simulink model "sm_boom_lift_crawler"  (R2026a)
settings: Solver=ode23t  StopTime=tVec.StopTime  FixedStep=2e-3  MaxStep=2  AbsTol=1e-3
StartFcn:
  | tic;
StopFcn:
  | Elapsed_Sim_Time = toc;
  | %disp(['Elapsed Sim Time = ' num2str(Elapsed_Sim_Time)]);
undefined symbols (not defined in the file): BasketR, Boom, Chassis, Extend, Jib, LevelM, LevelS, Lift, operator_seq, OutFL, OutFR, OutRL, OutRR, oVec, Tilt, TrackL, TrackR, Turret, tVec
libraries: sm_boom_lift_crawler_lib x14, nesl_utility x2, sm_lib x2, sm_boom_lift_crawler_lib_actuators x1, sm_boom_lift_crawler_lib_control x1, sm_boom_lift_crawler_lib_lift x1
(part 2 of 2)

== system sm_boom_lift_crawler/Control/Valve Sequence/Sky Valve Commands/Basket LevelS Selector Valve ==
  t : Inport
  Selector Valve Input : Lookup_n-D  NumberOfTableDimensions=1  BreakpointsForDimension1=[0 1]  Table=[0 0]  InterpMethod=Flat  ExtrapMethod=Clip  UseLastTableValue=on  InternalRulePriority=Speed  RndMeth=Simplest
  C : Outport
  wires:
  t/1 -> Selector Valve Input/1
  Selector Valve Input/1 -> C/1

== system sm_boom_lift_crawler/Control/Valve Sequence/Sky Valve Commands/BasketR Selector Valve (r2) ==
  t : Inport
  Selector Valve Input : Lookup_n-D  NumberOfTableDimensions=1  BreakpointsForDimension1=tVec.sky.r2.all  Table=oVec.sky.r2.all  InterpMethod=Flat  ExtrapMethod=Clip  UseLastTableValue=on  InternalRulePriority=Speed  RndMeth=Simplest
  C : Outport
  wires:
  Selector Valve Input/1 -> C/1
  t/1 -> Selector Valve Input/1

== system sm_boom_lift_crawler/Control/Valve Sequence/Sky Valve Commands/Extend Selector Valve (c3) ==
  t : Inport
  Selector Valve Input : Lookup_n-D  NumberOfTableDimensions=1  BreakpointsForDimension1=tVec.sky.c3.all  Table=oVec.sky.c3.all  InterpMethod=Flat  ExtrapMethod=Clip  UseLastTableValue=on  InternalRulePriority=Speed  RndMeth=Simplest
  C : Outport
  wires:
  t/1 -> Selector Valve Input/1
  Selector Valve Input/1 -> C/1

== system sm_boom_lift_crawler/Control/Valve Sequence/Sky Valve Commands/Jib Selector Valve (c4) ==
  t : Inport
  Selector Valve Input : Lookup_n-D  NumberOfTableDimensions=1  BreakpointsForDimension1=tVec.sky.c4.all  Table=oVec.sky.c4.all  InterpMethod=Flat  ExtrapMethod=Clip  UseLastTableValue=on  InternalRulePriority=Speed  RndMeth=Simplest
  C : Outport
  wires:
  Selector Valve Input/1 -> C/1
  t/1 -> Selector Valve Input/1

== system sm_boom_lift_crawler/Control/Valve Sequence/Sky Valve Commands/Lift Selector Valve (c1) ==
  t : Inport
  Selector Valve Input : Lookup_n-D  NumberOfTableDimensions=1  BreakpointsForDimension1=tVec.sky.c1.all  Table=oVec.sky.c1.all  InterpMethod=Flat  ExtrapMethod=Clip  UseLastTableValue=on  InternalRulePriority=Speed  RndMeth=Simplest
  C : Outport
  wires:
  t/1 -> Selector Valve Input/1
  Selector Valve Input/1 -> C/1

== system sm_boom_lift_crawler/Control/Valve Sequence/Sky Valve Commands/Sky Manifold Proportional Valve ==
  t : Inport
  Selector Valve Input : Lookup_n-D  NumberOfTableDimensions=1  BreakpointsForDimension1=tVec.sky.proportional  Table=oVec.sky.proportional  InterpMethod=Flat  ExtrapMethod=Clip  UseLastTableValue=on  InternalRulePriority=Speed  RndMeth=Simplest
  C : Outport
  wires:
  t/1 -> Selector Valve Input/1
  Selector Valve Input/1 -> C/1

== system sm_boom_lift_crawler/Control/Valve Sequence/Sky Valve Commands/Tilt Selector Valve (c2) ==
  t : Inport
  Selector Valve Input : Lookup_n-D  NumberOfTableDimensions=1  BreakpointsForDimension1=tVec.sky.c2.all  Table=oVec.sky.c2.all  InterpMethod=Flat  ExtrapMethod=Clip  UseLastTableValue=on  InternalRulePriority=Speed  RndMeth=Simplest
  C : Outport
  wires:
  Selector Valve Input/1 -> C/1
  t/1 -> Selector Valve Input/1

== system sm_boom_lift_crawler/Control/Valve Sequence/Sky Valve Commands/Turret Selector Valve (r1) ==
  t : Inport
  Selector Valve Input : Lookup_n-D  NumberOfTableDimensions=1  BreakpointsForDimension1=tVec.sky.r1.all  Table=oVec.sky.r1.all  InterpMethod=Flat  ExtrapMethod=Clip  UseLastTableValue=on  InternalRulePriority=Speed  RndMeth=Simplest
  C : Outport
  wires:
  t/1 -> Selector Valve Input/1
  Selector Valve Input/1 -> C/1
